simulink model "quad_equation_3d"  (R2024b)
settings: Solver=VariableStepAuto  StartTime=0.0  StopTime=2  RelTol=1e-3
values from neighbouring files (symbols this model uses):
  b_moment = 0.01    [quad_param_3d.m]
  g = 9.81    [quad_param_3d.m]
  I = [Ixx, 0, 0 ... (first row only)    [quad_param_3d.m]
  k = 0.01    [quad_param_3d.m]
  k_thrust = 0.1    [quad_param_3d.m]
  L = 0.086    [quad_param_3d.m]
  M = 3.3    [quad_param_3d.m]
  Xinit = [0;0;0;0;0;0;0;0;0;0;0;0]    [quad_param_3d.m]
libraries: simulink_extras x3
settings Model: Creator=Admin  LastModifiedBy=Admin

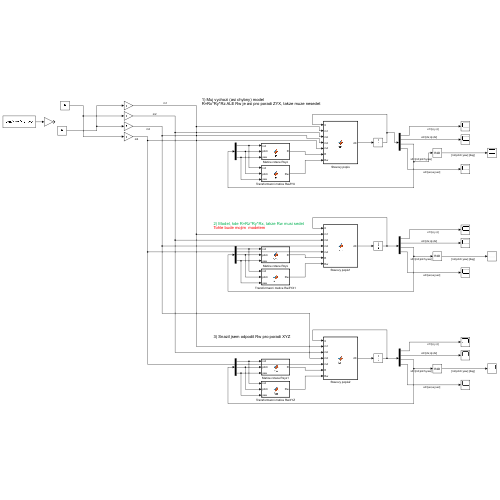
[thumbnail: Simulink's stored preview of the top-level diagram]
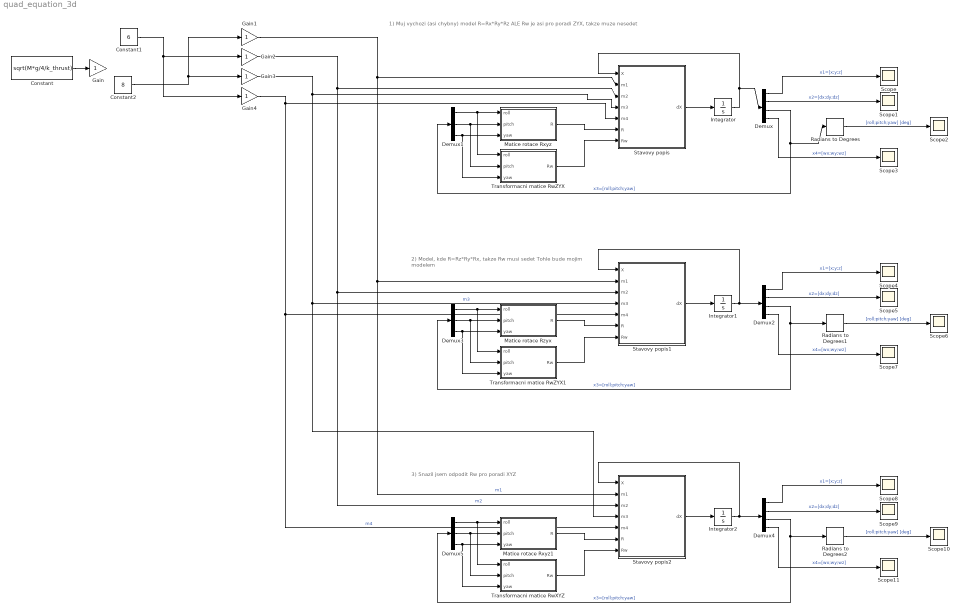
== system quad_equation_3d ==
  note: 1) Muj vychozi (asi chybny) model
      | R=Rx*Ry*Rz ALE Rw je asi pro poradi ZYX, takze muze nesedet
  note: 2) Model, kde R=Rz*Ry*Rx, takze Rw musi sedet
      | Tohle bude mojim modelem
  note: 3) Snazil jsem odpodit Rw pro poradi XYZ
  Constant : Constant  Value=sqrt(M*g/4/k_thrust)
  Constant1 : Constant  Value=6
  Constant2 : Constant  Value=8
  Demux : Demux
  Demux1 : Demux  Outputs=3
  Demux2 : Demux
  Demux3 : Demux  Outputs=3
  Demux4 : Demux
  Demux5 : Demux  Outputs=3
  Gain{,1..4} (5 alike) : Gain
  Integrator : Integrator  InitialCondition=Xinit
  Integrator1 : Integrator  InitialCondition=Xinit
  Integrator2 : Integrator  InitialCondition=Xinit
  Matice rotace Rxyz : MATLAB Function  TreatAsAtomicUnit=on
  Matice rotace Rxyz1 : MATLAB Function  TreatAsAtomicUnit=on
  Matice rotace Rzyx : MATLAB Function  TreatAsAtomicUnit=on
  Radians to Degrees : simulink_extras/Transformations/Radians to Degrees
  Radians to Degrees1 : simulink_extras/Transformations/Radians to Degrees
  Radians to Degrees2 : simulink_extras/Transformations/Radians to Degrees
  Scope{,1..11} (12 alike) : Scope
  Stavovy popis : MATLAB Function  TreatAsAtomicUnit=on
  Stavovy popis1 : MATLAB Function  TreatAsAtomicUnit=on
  Stavovy popis2 : MATLAB Function  TreatAsAtomicUnit=on
  Transformacni matice RwXYZ : MATLAB Function  TreatAsAtomicUnit=on
  Transformacni matice RwZYX : MATLAB Function  TreatAsAtomicUnit=on
  Transformacni matice RwZYX1 : MATLAB Function  TreatAsAtomicUnit=on
  wires:
  Matice rotace Rxyz/1(R) -> Stavovy popis/6(R)
  Transformacni matice RwZYX/1(Rw) -> Stavovy popis/7(Rw)
  Stavovy popis/1(dX) -> Integrator/1
  Integrator/1 -> Stavovy popis/1(X), Demux/1
  Demux/1 -> Scope/1  "x1=[x;y;z]"
  Demux/2 -> Scope1/1  "x2=[dx;dy;dz]"
  Demux/3 -> Radians to Degrees/1, Demux1/1  "x3=[roll;pitch;yaw]"
  Demux/4 -> Scope3/1  "x4=[wx;wy;wz]"
  Demux1/1 -> Transformacni matice RwZYX/1(roll), Matice rotace Rxyz/1(roll)
  Demux1/2 -> Matice rotace Rxyz/2(pitch), Transformacni matice RwZYX/2(pitch)
  Demux1/3 -> Matice rotace Rxyz/3(yaw), Transformacni matice RwZYX/3(yaw)
  Radians to Degrees/1 -> Scope2/1  "[roll;pitch;yaw] [deg]"
  Demux3/2 -> Matice rotace Rzyx/2(pitch), Transformacni matice RwZYX1/2(pitch)
  Demux3/3 -> Matice rotace Rzyx/3(yaw), Transformacni matice RwZYX1/3(yaw)
  Radians to Degrees1/1 -> Scope6/1  "[roll;pitch;yaw] [deg]"
  Transformacni matice RwZYX1/1(Rw) -> Stavovy popis1/7(Rw)
  Integrator1/1 -> Stavovy popis1/1(X), Demux2/1
  Stavovy popis1/1(dX) -> Integrator1/1
  Demux2/1 -> Scope4/1  "x1=[x;y;z]"
  Demux2/4 -> Scope7/1  "x4=[wx;wy;wz]"
  Demux2/2 -> Scope5/1  "x2=[dx;dy;dz]"
  Demux2/3 -> Radians to Degrees1/1, Demux3/1  "x3=[roll;pitch;yaw]"
  Matice rotace Rzyx/1(R) -> Stavovy popis1/6(R)
  Demux3/1 -> Transformacni matice RwZYX1/1(roll), Matice rotace Rzyx/1(roll)
  Constant/1 -> Gain/1
  Radians to Degrees2/1 -> Scope10/1  "[roll;pitch;yaw] [deg]"
  Demux5/2 -> Matice rotace Rxyz1/2(pitch), Transformacni matice RwXYZ/2(pitch)
  Integrator2/1 -> Stavovy popis2/1(X), Demux4/1
  Demux5/3 -> Matice rotace Rxyz1/3(yaw), Transformacni matice RwXYZ/3(yaw)
  Transformacni matice RwXYZ/1(Rw) -> Stavovy popis2/7(Rw)
  Demux5/1 -> Transformacni matice RwXYZ/1(roll), Matice rotace Rxyz1/1(roll)
  Demux4/3 -> Radians to Degrees2/1, Demux5/1  "x3=[roll;pitch;yaw]"
  Matice rotace Rxyz1/1(R) -> Stavovy popis2/6(R)
  Demux4/1 -> Scope8/1  "x1=[x;y;z]"
  Stavovy popis2/1(dX) -> Integrator2/1
  Demux4/2 -> Scope9/1  "x2=[dx;dy;dz]"
  Demux4/4 -> Scope11/1  "x4=[wx;wy;wz]"
  Gain1/1 -> Stavovy popis2/2(m1), Stavovy popis1/2(m1), Stavovy popis/2(m1)  "m1"
  Gain2/1 -> Stavovy popis2/3(m2), Stavovy popis1/3(m2), Stavovy popis/3(m2)  "m2"
  Gain3/1 -> Stavovy popis2/4(m3), Stavovy popis1/4(m3), Stavovy popis/4(m3)  "m3"
  Gain4/1 -> Stavovy popis2/5(m4), Stavovy popis1/5(m4), Stavovy popis/5(m4)  "m4"
  Constant2/1 -> Gain3/1, Gain1/1
  Constant1/1 -> Gain4/1, Gain2/1

== matlab function quad_equation_3d/Stavovy popis2 ==
  data: X input; m1 input; dX output; m2 input; m3 input; m4 input; R input; Rw input; k_thrust parameter; k parameter; I parameter; g parameter; M parameter; L parameter; b_moment parameter
function dX  = fcn(X, m1, m2, m3, m4, R, Rw, k_thrust, k, I, g, M, L, b_moment)
% m1, m2, m3, m4 jsou odpovidajici uhlove rychlosti rotoru
% Stavovy popis
% x1 - pozice dronu v prostoru, [x;y;z]
% x2 - linearni rychlost, [dx;dy;dz]
% x3 - Eulerove uhly, [roll;pitch;yaw]
% x4 - vektor uhlovych rychlosti, [wx;wy;wz]
x1 = X(1:3);
x2 = X(4:6);
x3 = X(7:9);
x4 = X(10:12);

Thrust = k_thrust*(m1^2 + m2^2 + m3^2 + m4^2); % tahova sila v soustave tela
Friction = -k * x2; % odporova sila v soustave sveta
Tau_roll = L*k_thrust*(m1^2 + m4^2 - m2^2 - m3^2);
Tau_pitch = L*k_thrust*(m4^2 + m3^2 - m1^2 - m2^2);
Tau_yaw = b_moment*(m1^2 + m3^2 - m2^2 - m4^2);

dx1 = x2;
dx2 = [0; 0; -g] + 1/M*R*[0; 0; Thrust] + 1/M*Friction;
dx3 = Rw \ x4;
dx4 = I\( [Tau_roll; Tau_pitch; Tau_yaw] -  cross( x4, (I*x4) ) );

dX = [dx1; dx2; dx3; dx4];

== matlab function quad_equation_3d/Transformacni matice RwXYZ ==
  data: roll input; Rw output; pitch input; yaw input
function Rw = fcn(roll, pitch, yaw)
% Prepocet matice pro transformace derivaci Eulerovych uhlu 
% do uhlove rychlosti v soustave tela ?

Rw = [cos(pitch)*cos(yaw), sin(yaw), 0;
     -cos(pitch)*sin(yaw), cos(yaw), 0;
      sin(pitch), 0, 1];

== matlab function quad_equation_3d/Matice rotace Rxyz ==
  data: roll input; R output; pitch input; yaw input
function R = fcn(roll, pitch, yaw)
% Prepocet matice rotace R=Rx*Ry*Rz

R_x = [1, 0, 0; 
       0, cos(roll), -sin(roll);
       0, sin(roll), cos(roll)];

R_y = [cos(pitch), 0, sin(pitch); 
       0, 1, 0; 
      -sin(pitch), 0, cos(pitch)];

R_z = [cos(yaw), -sin(yaw), 0; 
       sin(yaw), cos(yaw), 0; 
       0, 0, 1];

R = R_x * R_y * R_z;

== matlab function quad_equation_3d/Stavovy popis ==
  data: X input; m1 input; dX output; m2 input; m3 input; m4 input; R input; Rw input; k_thrust parameter; k parameter; I parameter; g parameter; M parameter; L parameter; b_moment parameter
function dX  = fcn(X, m1, m2, m3, m4, R, Rw, k_thrust, k, I, g, M, L, b_moment)
% m1, m2, m3, m4 jsou odpovidajici uhlove rychlosti rotoru
% Stavovy popis
% x1 - pozice dronu v prostoru, [x;y;z]
% x2 - linearni rychlost, [dx;dy;dz]
% x3 - Eulerove uhly, [roll;pitch;yaw]
% x4 - vektor uhlovych rychlosti, [wx;wy;wz]
x1 = X(1:3);
x2 = X(4:6);
x3 = X(7:9);
x4 = X(10:12);

Thrust = k_thrust*(m1^2 + m2^2 + m3^2 + m4^2); % tahova sila v soustave tela
Friction = -k * x2; % odporova sila v soustave sveta
Tau_roll = L*k_thrust*(m1^2 + m4^2 - m2^2 - m3^2);
Tau_pitch = L*k_thrust*(m4^2 + m3^2 - m1^2 - m2^2);
Tau_yaw = b_moment*(m1^2 + m3^2 - m2^2 - m4^2);

dx1 = x2;
dx2 = [0; 0; -g] + 1/M*R*[0; 0; Thrust] + 1/M*Friction;
dx3 = Rw \ x4;
dx4 = I\( [Tau_roll; Tau_pitch; Tau_yaw] -  cross( x4, (I*x4) ) );

dX = [dx1; dx2; dx3; dx4];

== matlab function quad_equation_3d/Transformacni matice RwZYX ==
  data: roll input; Rw output; pitch input; yaw input
function Rw = fcn(roll, pitch, yaw)
% Prepocet matice pro transformace derivaci Eulerovych uhlu 
% do uhlove rychlosti v soustave tela ?
Rw = [1, 0, -sin(pitch);
      0, cos(roll), cos(pitch)*sin(roll);
      0 -sin(roll), cos(pitch)*cos(roll)];

== matlab function quad_equation_3d/Matice rotace Rzyx ==
  data: roll input; R output; pitch input; yaw input
function R = fcn(roll, pitch, yaw)
% Prepocet matice rotace R=Rx*Ry*Rz

R_x = [1, 0, 0; 
       0, cos(roll), -sin(roll);
       0, sin(roll), cos(roll)];

R_y = [cos(pitch), 0, sin(pitch); 
       0, 1, 0; 
      -sin(pitch), 0, cos(pitch)];

R_z = [cos(yaw), -sin(yaw), 0; 
       sin(yaw), cos(yaw), 0; 
       0, 0, 1];

R = R_z * R_y * R_x;

== matlab function quad_equation_3d/Stavovy popis1 ==
  data: X input; m1 input; dX output; m2 input; m3 input; m4 input; R input; Rw input; k_thrust parameter; k parameter; I parameter; g parameter; M parameter; L parameter; b_moment parameter
function dX  = fcn(X, m1, m2, m3, m4, R, Rw, k_thrust, k, I, g, M, L, b_moment)
% m1, m2, m3, m4 jsou odpovidajici uhlove rychlosti rotoru
% Stavovy popis
% x1 - pozice dronu v prostoru, [x;y;z]
% x2 - linearni rychlost, [dx;dy;dz]
% x3 - Eulerove uhly, [roll;pitch;yaw]
% x4 - vektor uhlovych rychlosti, [wx;wy;wz]
x1 = X(1:3);
x2 = X(4:6);
x3 = X(7:9);
x4 = X(10:12);

Thrust = k_thrust*(m1^2 + m2^2 + m3^2 + m4^2); % tahova sila v soustave tela
Friction = -k * x2; % odporova sila v soustave sveta
Tau_roll = L*k_thrust*(m1^2 + m4^2 - m2^2 - m3^2);
Tau_pitch = L*k_thrust*(m4^2 + m3^2 - m1^2 - m2^2);
Tau_yaw = b_moment*(m1^2 + m3^2 - m2^2 - m4^2);

dx1 = x2;
dx2 = [0; 0; -g] + 1/M*R*[0; 0; Thrust] + 1/M*Friction;
dx3 = Rw \ x4;
dx4 = I\( [Tau_roll; Tau_pitch; Tau_yaw] -  cross( x4, (I*x4) ) );

dX = [dx1; dx2; dx3; dx4];

== matlab function quad_equation_3d/Transformacni matice RwZYX1 ==
  data: roll input; Rw output; pitch input; yaw input
function Rw = fcn(roll, pitch, yaw)
% Prepocet matice pro transformace derivaci Eulerovych uhlu 
% do uhlove rychlosti v soustave tela ?
Rw = [1, 0, -sin(pitch);
      0, cos(roll), cos(pitch)*sin(roll);
      0 -sin(roll), cos(pitch)*cos(roll)];

== matlab function quad_equation_3d/Matice rotace Rxyz1 ==
  data: roll input; R output; pitch input; yaw input
function R = fcn(roll, pitch, yaw)
% Prepocet matice rotace R=Rx*Ry*Rz

R_x = [1, 0, 0; 
       0, cos(roll), -sin(roll);
       0, sin(roll), cos(roll)];

R_y = [cos(pitch), 0, sin(pitch); 
       0, 1, 0; 
      -sin(pitch), 0, cos(pitch)];

R_z = [cos(yaw), -sin(yaw), 0; 
       sin(yaw), cos(yaw), 0; 
       0, 0, 1];

R = R_x * R_y * R_z;
